simulink library "Custom_Valve_Choices_Lib"  (R2013a)
settings: Solver=ode45  SolverMode=SingleTasking  StartTime=0.0  StopTime=10.0  RelTol=1e-3
libraries: fl_lib x57, sh_lib x10, nesl_utility x8, Custom_Valve_Orifices_Lib x3, Custom_Valve_Choices_Lib x1
(part 1 of 2)
Description:
  | Copyright 2013 The MathWorks, Inc.
settings Model: Creator=smiller  LastModifiedBy=smiller

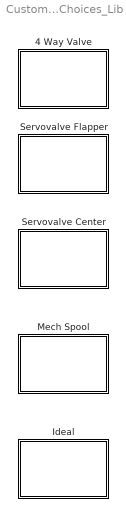
== system Custom_Valve_Choices_Lib ==
  4 Way Valve : Subsystem  BlockChoice=Ideal
      settings: TemplateBlock=self  MemberBlocks=Ideal,Mech Spool,Servovalve Center,Servovalve Flapper
      mask Display: disp(' ');
  Ideal : Subsystem  mask(Four-Way Valve){orifice_width=24.5, max_spool_travel=0.005, x0_orifice_PA=0, x0_orifice_PB=0, x0_orifice_AT=0, x0_orifice_BT=0}
      mask prompts: orifice_width "Orifice Width (mm):"; max_spool_travel "Max Orifice Length (m):"; x0_orifice_PA "Initial Opening PA (mm):"; x0_orifice_PB "Initial Opening PB (mm):"; x0_orifice_AT "Initial Opening AT (mm):"; x0_orifice_BT "Initial Opening BT (mm):"
      mask help: Four-way hydraulic directional valve.
      mask Display:
      | plot([0;337.311462499201;337.311462499201;0;0], [566.910021007061;566.910021007061;0;0;566.910021007061])
      | %hold on
      | plot([84.6585631370544;241.503668949008], [353;353])
      | plot([84.6585631370544;241.503668949008], [214;214])
      | plot([84.6585631370544;241.503668949008;241.503668949008;84.6585631370544;84.6585631370544], [491;491;76;76;491])
      | plot([84.6585631370544;241.503668949008], [449;449])
      | plot([241.503668949008;210.071657784283], [310;310])
      | plot([210.071657784283;210.071657784283;210.071657784283], [326;295;310.414731502533])
      | plot([241.503668949008;210.071657784283], [257;257])
      | plot([210.071657784283;210.071657784283;210.071657784283], [272;241;236.464468762279])
      | plot([84.6585631370544;115.964594297111], [257;257])
      | plot([115.964594297111;115.964594297111;115.964594297111], [272;241;236.464468762279])
      | plot([84.6585631370544;115.964594297111], [310;310])
      | plot([115.964594297111;115.964594297111;115.964594297111], [326;295;310.414731502533])
      | plot([84.6585631370544;241.503668949008], [185;110])
      | plot([241.503668949008;84.6585631370544], [185;110])
      | plot([84.6585631370544;241.503668949008], [395;395])
      | patch([85.0365031510592;110.547454096377;121.885654516518;85.0365031510592], [110;140;120;110], [0;0;0])
      | plot([85.0365031510592;110.547454096377;121.885654516518;85.0365031510592], [110;140;120;110])
      | patch([240.936758928001;204.087607562542;215.425807982683;240.936758928001], [109;120;140;109], [0;0;0])
      | plot([240.936758928001;204.087607562542;215.425807982683;240.936758928001], [109;120;140;109])
      | patch([83.6507230997086;127.554754726589;127.554754726589;83.6507230997086], [451;461;440;451], [0;0;0])
      | plot([83.6507230997086;127.554754726589;127.554754726589;83.6507230997086], [451;461;440;451])
      | patch([245.283069089055;201.253057457507;201.253057457507;245.283069089055], [394;405;384;394], [0;0;0])
      | plot([245.283069089055;201.253057457507;201.253057457507;245.283069089055], [394;405;384;394])
      | 
      | %plot([241.5; 241.5;201; 201], [491; 566; 566; 491])
      | %patch([241; 205; 222; 241], [525;525;495;525], [0;0;0]')
      | %plot([241.5; 241.5;201; 201], [76; 0; 0; 76])
      | %patch([241; 205; 222; 241], [40;40;70;40], [0;0;0])
      | %plot([241.5; 201], [11; 26])
      | %plot([241.5; 201], [561; 541])
      | 
      | %plot([127; 85;127; 85], [491; 511; 531; 551])
      | %plot([127; 85;127; 85], [76; 56; 36; 16])
      | %hold off
      | 
      | 
      | color('red');
      | port_label('LConn', 1,'A')
      | port_label('LConn', 2,'B')
      | port_label('RConn', 1,'S')
      | port_label('RConn', 2,'P')
      | port_label('RConn', 3,'T')
  Mech Spool : Subsystem  mask(Four-Way Valve with Spool){orifice_width=24.5, max_spool_travel=0.005, x0_orifice_PA=0, x0_orifice_PB=0, x0_orifice_AT=0, x0_orifice_BT=0, spool_mass=0.124, ctr_spr_stiffness=36000*100, spool_damping=324*10, spool_rad_clear=0.05}
      mask prompts: orifice_width "Orifice Width (mm):"; max_spool_travel "Max Orifice Length (m):"; x0_orifice_PA "Initial Opening PA (mm):"; x0_orifice_PB "Initial Opening PB (mm):"; x0_orifice_AT "Initial Opening AT (mm):"; x0_orifice_BT "Initial Opening BT (mm):"; spool_mass "Spool Mass (kg):"; ctr_spr_stiffness "Centering Spring Stiffness (N/m):"; spool_damping "Spool Damping (N/(m/s)):"; spool_rad_clear "Spool Radial Clearance (mm):"
      mask help: Four-way valve including mechanical model of spool. The spool is centered by a spring.
      mask Display:
      | plot([0;337.311462499201;337.311462499201;0;0], [566.910021007061;566.910021007061;0;0;566.910021007061])
      | %hold on
      | plot([84.6585631370544;241.503668949008], [353;353])
      | plot([84.6585631370544;241.503668949008], [214;214])
      | plot([84.6585631370544;241.503668949008;241.503668949008;84.6585631370544;84.6585631370544], [491;491;76;76;491])
      | plot([84.6585631370544;241.503668949008], [449;449])
      | plot([241.503668949008;210.071657784283], [310;310])
      | plot([210.071657784283;210.071657784283;210.071657784283], [326;295;310.414731502533])
      | plot([241.503668949008;210.071657784283], [257;257])
      | plot([210.071657784283;210.071657784283;210.071657784283], [272;241;236.464468762279])
      | plot([84.6585631370544;115.964594297111], [257;257])
      | plot([115.964594297111;115.964594297111;115.964594297111], [272;241;236.464468762279])
      | plot([84.6585631370544;115.964594297111], [310;310])
      | plot([115.964594297111;115.964594297111;115.964594297111], [326;295;310.414731502533])
      | plot([84.6585631370544;241.503668949008], [185;110])
      | plot([241.503668949008;84.6585631370544], [185;110])
      | plot([84.6585631370544;241.503668949008], [395;395])
      | patch([85.0365031510592;110.547454096377;121.885654516518;85.0365031510592], [110;140;120;110], [0;0;0])
      | plot([85.0365031510592;110.547454096377;121.885654516518;85.0365031510592], [110;140;120;110])
      | patch([240.936758928001;204.087607562542;215.425807982683;240.936758928001], [109;120;140;109], [0;0;0])
      | plot([240.936758928001;204.087607562542;215.425807982683;240.936758928001], [109;120;140;109])
      | patch([83.6507230997086;127.554754726589;127.554754726589;83.6507230997086], [451;461;440;451], [0;0;0])
      | plot([83.6507230997086;127.554754726589;127.554754726589;83.6507230997086], [451;461;440;451])
      | patch([245.283069089055;201.253057457507;201.253057457507;245.283069089055], [394;405;384;394], [0;0;0])
      | plot([245.283069089055;201.253057457507;201.253057457507;245.283069089055], [394;405;384;394])
      | 
      | plot([241.5; 241.5;201; 201], [491; 566; 566; 491])
      | %patch([241; 205; 222; 241], [525;525;495;525], [0;0;0]')
      | plot([241.5; 241.5;201; 201], [76; 0; 0; 76])
      | %patch([241; 205; 222; 241], [40;40;70;40], [0;0;0])
      | %plot([241.5; 201], [11; 26])
      | %plot([241.5; 201], [561; 541])
      | 
      | plot([127; 85;127; 85], [491; 511; 531; 551])
      | plot([127; 85;127; 85], [76; 56; 36; 16])
      | %hold off
      | 
      | 
      | color('cyan');
      | port_label('LConn', 1,'A')
      | port_label('LConn', 2,'B')
      | port_label('RConn', 1,'S')
      | port_label('RConn', 2,'P')
      | port_label('RConn', 3,'T')
  Servovalve Center : Subsystem  mask(Four-Way Servovalve, Centering Spring){orifice_width=24.5, max_spool_travel=0.005, x0_orifice_PA=0, x0_orifice_PB=0, x0_orifice_AT=0, x0_orifice_BT=0, spool_mass=0.124, ctr_spr_stiffness=3600000, spool_damping=162, spool_rad_clear=0.05, x0_nozzle=0.5, max_nozzle_area=3.14, pump_spool_orifice_area=1}
      mask prompts: orifice_width "Orifice Width (mm):"; max_spool_travel "Max Orifice Length (m):"; x0_orifice_PA "Initial Opening PA (mm):"; x0_orifice_PB "Initial Opening PB (mm):"; x0_orifice_AT "Initial Opening AT (mm):"; x0_orifice_BT "Initial Opening BT (mm):"; spool_mass "Spool Mass (kg):"; ctr_spr_stiffness "Centering Spring Stiffness (N/m):"; spool_damping "Spool Damping (N/(m/s)):"; spool_rad_clear "Spool Radial Clearance (mm):"; x0_nozzle "Nozzle Initial Opening (mm):"; max_nozzle_area "Nozzle Max Area (mm^2):"; pump_spool_orifice_area "Pump Spool Orifice Area (mm^2):"
      mask help: Four-way servovalve with electrical actuation of a flapper nozzle to control spool movement. The spool is centered by a spring.
      mask Display:
      | plot([0;337.311462499201;337.311462499201;0;0], [566.910021007061;566.910021007061;0;0;566.910021007061])
      | %hold on
      | plot([84.6585631370544;241.503668949008], [353;353])
      | plot([84.6585631370544;241.503668949008], [214;214])
      | plot([84.6585631370544;241.503668949008;241.503668949008;84.6585631370544;84.6585631370544], [491;491;76;76;491])
      | plot([84.6585631370544;241.503668949008], [449;449])
      | plot([241.503668949008;210.071657784283], [310;310])
      | plot([210.071657784283;210.071657784283;210.071657784283], [326;295;310.414731502533])
      | plot([241.503668949008;210.071657784283], [257;257])
      | plot([210.071657784283;210.071657784283;210.071657784283], [272;241;236.464468762279])
      | plot([84.6585631370544;115.964594297111], [257;257])
      | plot([115.964594297111;115.964594297111;115.964594297111], [272;241;236.464468762279])
      | plot([84.6585631370544;115.964594297111], [310;310])
      | plot([115.964594297111;115.964594297111;115.964594297111], [326;295;310.414731502533])
      | plot([84.6585631370544;241.503668949008], [185;110])
      | plot([241.503668949008;84.6585631370544], [185;110])
      | plot([84.6585631370544;241.503668949008], [395;395])
      | patch([85.0365031510592;110.547454096377;121.885654516518;85.0365031510592], [110;140;120;110], [0;0;0])
      | plot([85.0365031510592;110.547454096377;121.885654516518;85.0365031510592], [110;140;120;110])
      | patch([240.936758928001;204.087607562542;215.425807982683;240.936758928001], [109;120;140;109], [0;0;0])
      | plot([240.936758928001;204.087607562542;215.425807982683;240.936758928001], [109;120;140;109])
      | patch([83.6507230997086;127.554754726589;127.554754726589;83.6507230997086], [451;461;440;451], [0;0;0])
      | plot([83.6507230997086;127.554754726589;127.554754726589;83.6507230997086], [451;461;440;451])
      | patch([245.283069089055;201.253057457507;201.253057457507;245.283069089055], [394;405;384;394], [0;0;0])
      | plot([245.283069089055;201.253057457507;201.253057457507;245.283069089055], [394;405;384;394])
      | 
      | plot([241.5; 241.5;201; 201], [491; 566; 566; 491])
      | patch([241; 205; 222; 241], [525;525;495;525], [0;0;0]')
      | plot([241.5; 241.5;201; 201], [76; 0; 0; 76])
      | patch([241; 205; 222; 241], [40;40;70;40], [0;0;0])
      | %plot([241.5; 201], [11; 26])
      | %plot([241.5; 201], [561; 541])
      | 
      | plot([127; 85;127; 85], [491; 511; 531; 551])
      | plot([127; 85;127; 85], [76; 56; 36; 16])
      | %hold off
      | 
      | ;color('orange');
      | port_label('LConn', 1,'A')
      | port_label('LConn', 2,'B')
      | port_label('RConn', 1,'S')
      | port_label('RConn', 2,'P')
      | port_label('RConn', 3,'T')
  Servovalve Flapper : Subsystem  mask(Four-Way Servovalve, Flapper-Spool){orifice_width=24.5, max_spool_travel=0.005, x0_orifice_PA=0, x0_orifice_PB=0, x0_orifice_AT=0, x0_orifice_BT=0, spool_mass=0.124, spool_damping=162, spool_rad_clear=0.05, x0_nozzle=0.5, max_nozzle_area=3.14, pump_spool_orifice_area=1}
      mask prompts: orifice_width "Orifice Width (mm):"; max_spool_travel "Max Orifice Length (m):"; x0_orifice_PA "Initial Opening PA (mm):"; x0_orifice_PB "Initial Opening PB (mm):"; x0_orifice_AT "Initial Opening AT (mm):"; x0_orifice_BT "Initial Opening BT (mm):"; spool_mass "Spool Mass (kg):"; spool_damping "Centering Spring Damping (N/(m/s)):"; spool_rad_clear "Spool Radial Clearance (mm):"; x0_nozzle "Nozzle Initial Opening (mm):"; max_nozzle_area "Nozzle Max Area (mm^2):"; pump_spool_orifice_area "Pump Spool Orifice Area (mm):"
      mask help: Four-way servovalve with electrical actuation of a flapper-nozzle to control spool movement. The flapper is connected mechanically to spool.
      mask Display:
      | plot([0;337.311462499201;337.311462499201;0;0], [566.910021007061;566.910021007061;0;0;566.910021007061])
      | %hold on
      | plot([84.6585631370544;241.503668949008], [353;353])
      | plot([84.6585631370544;241.503668949008], [214;214])
      | plot([84.6585631370544;241.503668949008;241.503668949008;84.6585631370544;84.6585631370544], [491;491;76;76;491])
      | plot([84.6585631370544;241.503668949008], [449;449])
      | plot([241.503668949008;210.071657784283], [310;310])
      | plot([210.071657784283;210.071657784283;210.071657784283], [326;295;310.414731502533])
      | plot([241.503668949008;210.071657784283], [257;257])
      | plot([210.071657784283;210.071657784283;210.071657784283], [272;241;236.464468762279])
      | plot([84.6585631370544;115.964594297111], [257;257])
      | plot([115.964594297111;115.964594297111;115.964594297111], [272;241;236.464468762279])
      | plot([84.6585631370544;115.964594297111], [310;310])
      | plot([115.964594297111;115.964594297111;115.964594297111], [326;295;310.414731502533])
      | plot([84.6585631370544;241.503668949008], [185;110])
      | plot([241.503668949008;84.6585631370544], [185;110])
      | plot([84.6585631370544;241.503668949008], [395;395])
      | patch([85.0365031510592;110.547454096377;121.885654516518;85.0365031510592], [110;140;120;110], [0;0;0])
      | plot([85.0365031510592;110.547454096377;121.885654516518;85.0365031510592], [110;140;120;110])
      | patch([240.936758928001;204.087607562542;215.425807982683;240.936758928001], [109;120;140;109], [0;0;0])
      | plot([240.936758928001;204.087607562542;215.425807982683;240.936758928001], [109;120;140;109])
      | patch([83.6507230997086;127.554754726589;127.554754726589;83.6507230997086], [451;461;440;451], [0;0;0])
      | plot([83.6507230997086;127.554754726589;127.554754726589;83.6507230997086], [451;461;440;451])
      | patch([245.283069089055;201.253057457507;201.253057457507;245.283069089055], [394;405;384;394], [0;0;0])
      | plot([245.283069089055;201.253057457507;201.253057457507;245.283069089055], [394;405;384;394])
      | 
      | plot([241.5; 241.5;201; 201], [491; 566; 566; 491])
      | patch([241; 205; 222; 241], [525;525;495;525], [0;0;0]')
      | plot([241.5; 241.5;201; 201], [76; 0; 0; 76])
      | patch([241; 205; 222; 241], [40;40;70;40], [0;0;0])
      | %plot([241.5; 201], [11; 26])
      | %plot([241.5; 201], [561; 541])
      | 
      | %plot([127; 85;127; 85], [491; 511; 531; 551])
      | %plot([127; 85;127; 85], [76; 56; 36; 16])
      | %hold off
      | 
      | 
      | color('green');
      | port_label('LConn', 1,'A')
      | port_label('LConn', 2,'B')
      | port_label('RConn', 1,'S')
      | port_label('RConn', 2,'P')
      | port_label('RConn', 3,'T')

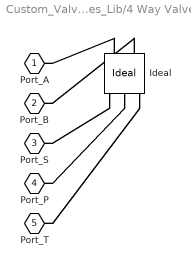
== system Custom_Valve_Choices_Lib/4 Way Valve ==
  Ideal : Custom_Valve_Choices_Lib/Ideal  orifice_width=24.5  max_spool_travel=0.005  x0_orifice_PA=0  x0_orifice_PB=0  x0_orifice_AT=0  x0_orifice_BT=0
  Port_A : PMIOPort  Port=1  Side=Left
  Port_B : PMIOPort  Port=2  Side=Left
  Port_S : PMIOPort  Port=3  Side=Right
  Port_P : PMIOPort  Port=4  Side=Right
  Port_T : PMIOPort  Port=5  Side=Right
  connections:
  Ideal/LConn1 -- Port_A/RConn1
  Ideal/LConn2 -- Port_B/RConn1
  Ideal/RConn1 -- Port_S/RConn1
  Ideal/RConn2 -- Port_P/RConn1
  Ideal/RConn3 -- Port_T/RConn1

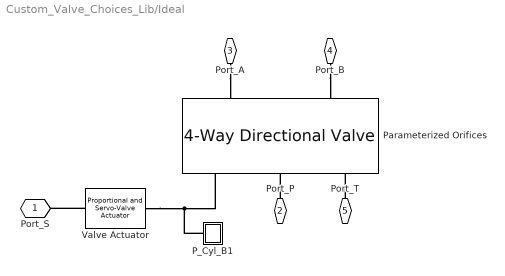
== system Custom_Valve_Choices_Lib/Ideal ==
  P_Cyl_B1 : Subsystem
  Parameterized Orifices : sh_lib/Valves/Directional Valves/4-Way Directional Valve  mdl_type=1  area_max=orifice_width*max_spool_travel*1e3 mm^2  opening_max=max_spool_travel m  opening_tab="[  -0.002 0 0.002 0.005 0.015 ] m"  area_tab="[  1e-09 2.0352e-07 4.0736e-05 0.00011438 0.00034356 ] m^2"  pressure_tab="[  -1e+07 -5e+06 -2e+06 2e+06 5e+06 1e+07 ] Pa"  flow_rate_tab="[  -1e-07 -7.0711e-08 -4.4721e-08 4.4721e-08 7.0711e-08 1e-07 ; -2.0352e-05 -1.4391e-05 -9.1017e-06 9.1017e-06 1.4391e-05 2.0352e-05 ; -0.0040736 -0.0028805 -0.0018218 0.0018218 0.0028805 0.0040736 ; -0.011438 -0.0080879 -0.0051152 0.0051152 0.0080879 0.011438 ; -0.034356 -0.024293 -0.015364 0.015364 0.024293 0.034356 ; ] m^3/s"  interp_method=1  extrap_method=1  C_d=0.7  x_0_P_A=x0_orifice_PA mm  x_0_P_B=x0_orifice_PB mm  x_0_A_T=x0_orifice_AT mm  x_0_B_T=x0_orifice_BT mm  Re_cr=12  A_leak=1e-12 m^2  LocalVarLogging=[]
  Valve Actuator : sh_lib/Valves/Valve Actuators/Proportional and Servo-Valve Actuator  gain=250  time_constant=1e-2 s  saturation=0.3  LocalVarLogging=[]
  Port_S : PMIOPort  Port=1  Side=Right
  Port_P : PMIOPort  Port=2  Side=Right
  Port_A : PMIOPort  Port=3  Side=Left
  Port_B : PMIOPort  Port=4  Side=Left
  Port_T : PMIOPort  Port=5  Side=Right
  connections:
  Valve Actuator/LConn1 -- Port_S/RConn1
  Port_T/RConn1 -- Parameterized Orifices/RConn3
  Port_P/RConn1 -- Parameterized Orifices/RConn2
  Parameterized Orifices/RConn1 -- P_Cyl_B1/LConn1 -- Valve Actuator/RConn1
  Port_B/RConn1 -- Parameterized Orifices/LConn2
  Port_A/RConn1 -- Parameterized Orifices/LConn1

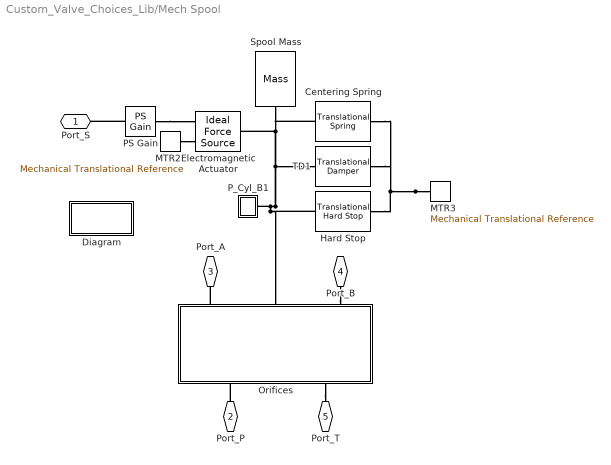
== system Custom_Valve_Choices_Lib/Mech Spool ==
  Centering Spring : fl_lib/Mechanical/Translational Elements/Translational Spring  Tag=Factory Generic  spr_rate=ctr_spr_stiffness N/m  init_def=0 m  f_Log=off  v_Log=off  x_Log=off  LocalVarNames=|force|deformation  LocalVarDescs=|Spring force (N)|Spring deformation (m)  LocalVarLogging=[0 0]
  Diagram : Subsystem
      mask Display: image(imread('Custom_Valve_Proportional_Spool.jpg'));
  Electromagnetic Actuator : fl_lib/Mechanical/Mechanical Sources/Ideal Force Source  Tag=Factory Generic  v_Log=off  f_Log=off  LocalVarNames=|force|rel_velocity|power  LocalVarDescs=|Force (N)|Relative velocity (m/s)|Power generated by the source (W)  LocalVarLogging=[0 0 0]
  Hard Stop : fl_lib/Mechanical/Translational Elements/Translational Hard Stop  Tag=Factory Generic  upper_bnd=max_spool_travel m  lower_bnd=-max_spool_travel m  stiff_up=1e+06 N/m  stiff_low=1e+06 N/m  D_up=150 N/(m/s)  D_low=150 N/(m/s)  initial_position=0 m  f_Log=off  v_Log=off  x_Log=off  LocalVarNames=|contact_force|rel_displacement  LocalVarDescs=|Contact force (N)|Slider-case relative displacement (m)  LocalVarLogging=[0 0]
  MTR2 : fl_lib/Mechanical/Translational Elements/Mechanical Translational Reference  Tag=Factory Generic  f_Log=off  LocalVarNames=|f  LocalVarDescs=|f  LocalVarLogging=[]
  MTR3 : fl_lib/Mechanical/Translational Elements/Mechanical Translational Reference  Tag=Factory Generic  f_Log=off  LocalVarNames=|f  LocalVarDescs=|f  LocalVarLogging=[]
  Orifices : Subsystem  BlockChoice=No Force
      link override No Force: or_width=orifice_width  x0_PA=x0_orifice_PA  x0_PB=x0_orifice_PB  x0_AT=x0_orifice_AT  x0_BT=x0_orifice_BT
      link override Parameterized: or_width=orifice_width  x0_PA=x0_orifice_PA  x0_PB=x0_orifice_PA  x0_AT=x0_orifice_PA  x0_BT=x0_orifice_PA  max_sp_trv=max_spool_travel
      link override With Force: or_width=orifice_width  x0_PA=x0_orifice_PA  x0_PB=x0_orifice_PB  x0_AT=x0_orifice_AT  x0_BT=x0_orifice_BT  rad_clearance=spool_rad_clear
      settings: AttributesFormatString=%<BlockChoice>  TemplateBlock=Custom_Valve_Orifices_Lib/Orifices  MemberBlocks=No Force,Parameterized,With Force
  PS Gain : fl_lib/Physical Signals/Functions/PS Gain  gain=5e4*100  LocalVarLogging=[]
  P_Cyl_B1 : Subsystem
  Spool Mass : fl_lib/Mechanical/Translational Elements/Mass  Tag=Factory Generic  mass=spool_mass kg  initial_velocity=0 m/s  f_Log=off  LocalVarNames=|force|velocity  LocalVarDescs=|Inertia force (N)|Mass absolute velocity (m/s)  LocalVarLogging=[0 0]
  TD1 : fl_lib/Mechanical/Translational Elements/Translational Damper  Tag=Factory Generic  D=spool_damping N/(m/s)  f_Log=off  v_Log=off  LocalVarNames=|force|rel_velocity|power  LocalVarDescs=|Damping force (N)|Damper relative velocity (m/s)|Power dissipated in the damper (W)  LocalVarLogging=[0 0 0]
  Port_S : PMIOPort  Port=1  Side=Right
  Port_P : PMIOPort  Port=2  Side=Right
  Port_A : PMIOPort  Port=3  Side=Left
  Port_B : PMIOPort  Port=4  Side=Left
  Port_T : PMIOPort  Port=5  Side=Right
  connections:
  Port_P/RConn1 -- Orifices/LConn1
  Orifices/RConn1 -- Port_A/RConn1
  Port_B/RConn1 -- Orifices/RConn3
  P_Cyl_B1/LConn1 -- Electromagnetic Actuator/LConn1 -- Spool Mass/LConn1 -- Centering Spring/LConn1 -- TD1/LConn1 -- Hard Stop/LConn1 -- Orifices/RConn2
  Orifices/LConn2 -- Port_T/RConn1
  MTR3/LConn1 -- Hard Stop/RConn1 -- Centering Spring/RConn1 -- TD1/RConn1
  PS Gain/RConn1 -- Electromagnetic Actuator/RConn1
  PS Gain/LConn1 -- Port_S/RConn1
  MTR2/LConn1 -- Electromagnetic Actuator/RConn2

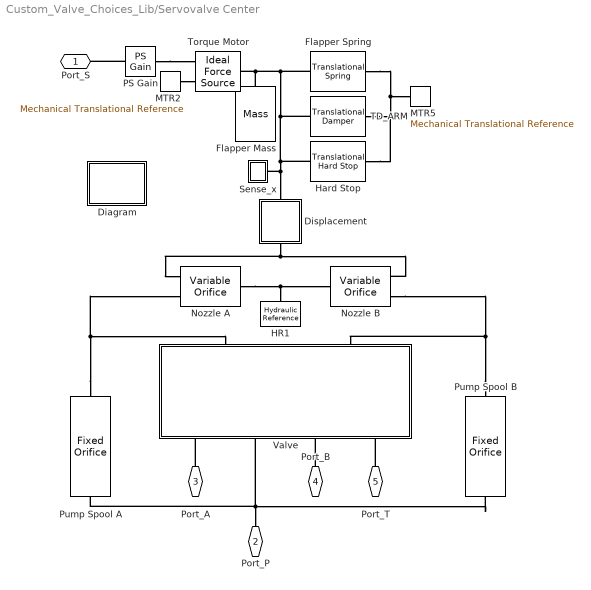
== system Custom_Valve_Choices_Lib/Servovalve Center ==
  Diagram : Subsystem
      mask Display: image(imread('Custom_Valve_Servovalve_Spring_Centered.jpg'));
  Displacement : Subsystem
      mask Display:
      | plot([311.800511553884;0;0;311.800511553884;311.800511553884], [311.800511553884;311.800511553884;0;0;311.800511553884])
      | plot([25.5109509453177;56.6910021007061;70.8637526258826;96.3747035712004;127.554754726589;155.900255776942;184.245756827295;212.591257877648;235.26765871793;252.274959348142;283.455010503531], [155.900255776942;155.900255776942;110.547454096377;198.418507352471;113.382004201412;198.418507352471;116.216554306448;198.418507352471;113.382004201412;155.900255776942;155.900255776942])
      | plot([155.900255776942;155.900255776942], [266.447709873319;198.418507352471])
      | patch([155.900255776942;170.073006302118;141.727505251765;155.900255776942], [198.418507352471;226.764008402824;226.764008402824;198.418507352471], [0;0;0])
      | plot([155.900255776942;170.073006302118;141.727505251765;155.900255776942], [198.418507352471;226.764008402824;226.764008402824;198.418507352471])
  Flapper Mass : fl_lib/Mechanical/Translational Elements/Mass  Tag=Factory Generic  mass=0.012 kg  initial_velocity=0 m/s  f_Log=off  LocalVarNames=|force|velocity  LocalVarDescs=|Inertia force (N)|Mass absolute velocity (m/s)  LocalVarLogging=[0 0]
  Flapper Spring : fl_lib/Mechanical/Translational Elements/Translational Spring  Tag=Factory Generic  spr_rate=150000 N/m  init_def=0 m  f_Log=off  v_Log=off  x_Log=off  LocalVarNames=|force|deformation  LocalVarDescs=|Spring force (N)|Spring deformation (m)  LocalVarLogging=[0 0]
  HR1 : fl_lib/Hydraulic/Hydraulic Elements/Hydraulic Reference  Tag=Factory Generic  q_Log=off  LocalVarNames=|q  LocalVarDescs=|q  LocalVarLogging=[]
  Hard Stop : fl_lib/Mechanical/Translational Elements/Translational Hard Stop  Tag=Factory Generic  upper_bnd=x0_nozzle mm  lower_bnd=-x0_nozzle mm  stiff_up=1e+06 N/m  stiff_low=1e+06 N/m  D_up=150 N/(m/s)  D_low=150 N/(m/s)  initial_position=0 m  f_Log=off  v_Log=off  x_Log=off  LocalVarNames=|contact_force|rel_displacement  LocalVarDescs=|Contact force (N)|Slider-case relative displacement (m)  LocalVarLogging=[0 0]
  MTR2 : fl_lib/Mechanical/Translational Elements/Mechanical Translational Reference  Tag=Factory Generic  f_Log=off  LocalVarNames=|f  LocalVarDescs=|f  LocalVarLogging=[]
  MTR5 : fl_lib/Mechanical/Translational Elements/Mechanical Translational Reference  Tag=Factory Generic  f_Log=off  LocalVarNames=|f  LocalVarDescs=|f  LocalVarLogging=[]
  Nozzle A : sh_lib/Orifices/Variable Orifice  Tag=Factory Generic  mdl_type=1  area_max=max_nozzle_area mm^2  opening_max=2*x0_nozzle mm  opening_tab="[  -0.002 0 0.005 0.015 ] m"  area_tab="[  1e-12 4e-12 1e-05 1.02e-05 ] m^2"  pressure_tab="[  -5e+06 -2e+06 2e+06 5e+06 ] Pa"  flow_rate_tab="[  -1e-12 -6e-14 6e+12 1e+11 ; -8e-08 -4e-08 4e+06 8e+06 ; -0.0025 -0.00103 0.001 0.0024 ; -0.00258 -0.001032 0.00106 0.00247 ; ] m^3/s"  interp_method=1  extrap_method=1  or=1  C_d=0.7  x_0=x0_nozzle mm  Re_cr=12  A_leak=1e-9 m^2  flow_rate_Log=off  pr_drop_Log=off  Re_Log=off  orif_opening_Log=off  power_Log=off  LocalVarNames=|flow_rate|pr_drop|Re|orif_opening|power  LocalVarDescs=|Flow rate through the orifice (m^3)|Pressure drop across the orifice (Pa)|Reynolds number|Orifice opening (m)|Power dissipated in the orifice (W)  LocalVarLogging=[0 0 0 0 0]
  Nozzle B : sh_lib/Orifices/Variable Orifice  Tag=Factory Generic  mdl_type=1  area_max=max_nozzle_area mm^2  opening_max=2*x0_nozzle mm  opening_tab="[  -0.002 0 0.005 0.015 ] m"  area_tab="[  1e-12 4e-12 1e-05 1.02e-05 ] m^2"  pressure_tab="[  -5e+06 -2e+06 2e+06 5e+06 ] Pa"  flow_rate_tab="[  -1e-12 -6e-14 6e+12 1e+11 ; -8e-08 -4e-08 4e+06 8e+06 ; -0.0025 -0.00103 0.001 0.0024 ; -0.00258 -0.001032 0.00106 0.00247 ; ] m^3/s"  interp_method=1  extrap_method=1  or=2  C_d=0.7  x_0=x0_nozzle mm  Re_cr=12  A_leak=1e-9 m^2  flow_rate_Log=off  pr_drop_Log=off  Re_Log=off  orif_opening_Log=off  power_Log=off  LocalVarNames=|flow_rate|pr_drop|Re|orif_opening|power  LocalVarDescs=|Flow rate through the orifice (m^3)|Pressure drop across the orifice (Pa)|Reynolds number|Orifice opening (m)|Power dissipated in the orifice (W)  LocalVarLogging=[0 0 0 0 0]
  PS Gain : fl_lib/Physical Signals/Functions/PS Gain  gain=-5e4  LocalVarLogging=[]
  "Pump Spool A " : sh_lib/Orifices/Fixed Orifice  Tag=Factory Generic  area=pump_spool_orifice_area mm^2  C_d=0.7  Re_cr=12  flow_rate_Log=off  pr_drop_Log=off  Re_Log=off  power_Log=off  LocalVarNames=|flow_rate|pr_drop|Re|power  LocalVarDescs=|Flow rate through the orifice (m^3/s)|Pressure drop across the orifice (Pa)|Reynolds number|Power (W)  LocalVarLogging=[0 0 0 0]
  Pump Spool B : sh_lib/Orifices/Fixed Orifice  Tag=Factory Generic  area=pump_spool_orifice_area mm^2  C_d=0.7  Re_cr=12  flow_rate_Log=off  pr_drop_Log=off  Re_Log=off  power_Log=off  LocalVarNames=|flow_rate|pr_drop|Re|power  LocalVarDescs=|Flow rate through the orifice (m^3/s)|Pressure drop across the orifice (Pa)|Reynolds number|Power (W)  LocalVarLogging=[0 0 0 0]
  Sense_x : Subsystem
  TD_ARM : fl_lib/Mechanical/Translational Elements/Translational Damper  Tag=Factory Generic  D=25 N/(m/s)  f_Log=off  v_Log=off  LocalVarNames=|force|rel_velocity|power  LocalVarDescs=|Damping force (N)|Damper relative velocity (m/s)|Power dissipated in the damper (W)  LocalVarLogging=[0 0 0]
  Torque Motor : fl_lib/Mechanical/Mechanical Sources/Ideal Force Source  Tag=Factory Generic  v_Log=off  f_Log=off  LocalVarNames=|force|rel_velocity|power  LocalVarDescs=|Force (N)|Relative velocity (m/s)|Power generated by the source (W)  LocalVarLogging=[0 0 0]
  Valve : Subsystem
  Port_S : PMIOPort  Port=1  Side=Right
  Port_P : PMIOPort  Port=2  Side=Right
  Port_A : PMIOPort  Port=3  Side=Left
  Port_B : PMIOPort  Port=4  Side=Left
  Port_T : PMIOPort  Port=5  Side=Right
  connections:
  Port_T/RConn1 -- Valve/RConn4
  Port_B/RConn1 -- Valve/RConn3
  Port_A/RConn1 -- Valve/RConn1
  PS Gain/RConn1 -- Torque Motor/RConn1
  PS Gain/LConn1 -- Port_S/RConn1
  Hard Stop/LConn1 -- Displacement/LConn1 -- Sense_x/LConn1 -- TD_ARM/LConn1 -- Flapper Spring/LConn1 -- Flapper Mass/LConn1 -- Torque Motor/LConn1
  Displacement/RConn1 -- Nozzle B/LConn1 -- Nozzle A/LConn1
  Pump Spool B/LConn1 -- "Pump Spool A "/LConn1 -- Port_P/RConn1 -- Valve/RConn2
  Flapper Spring/RConn1 -- MTR5/LConn1 -- Hard Stop/RConn1 -- TD_ARM/RConn1
  Nozzle A/RConn1 -- HR1/LConn1 -- Nozzle B/RConn1
  "Pump Spool A "/RConn1 -- Nozzle A/LConn2 -- Valve/LConn1
  Pump Spool B/RConn1 -- Nozzle B/LConn2 -- Valve/LConn2
  MTR2/LConn1 -- Torque Motor/RConn2

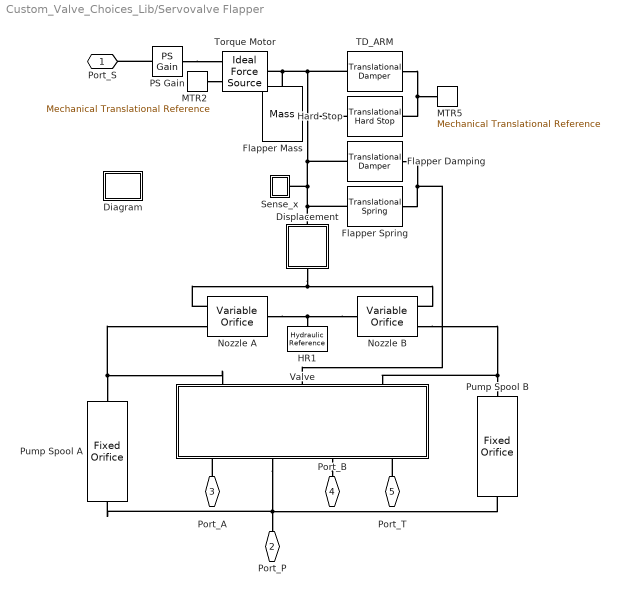
== system Custom_Valve_Choices_Lib/Servovalve Flapper ==
  Diagram : Subsystem
      mask Display: image(imread('Custom_Valve_Servovalve_Feedback.jpg'));
  Displacement : Subsystem
      mask Display:
      | plot([311.800511553884;0;0;311.800511553884;311.800511553884], [311.800511553884;311.800511553884;0;0;311.800511553884])
      | plot([25.5109509453177;56.6910021007061;70.8637526258826;96.3747035712004;127.554754726589;155.900255776942;184.245756827295;212.591257877648;235.26765871793;252.274959348142;283.455010503531], [155.900255776942;155.900255776942;110.547454096377;198.418507352471;113.382004201412;198.418507352471;116.216554306448;198.418507352471;113.382004201412;155.900255776942;155.900255776942])
      | plot([155.900255776942;155.900255776942], [266.447709873319;198.418507352471])
      | patch([155.900255776942;170.073006302118;141.727505251765;155.900255776942], [198.418507352471;226.764008402824;226.764008402824;198.418507352471], [0;0;0])
      | plot([155.900255776942;170.073006302118;141.727505251765;155.900255776942], [198.418507352471;226.764008402824;226.764008402824;198.418507352471])
  Flapper Damping : fl_lib/Mechanical/Translational Elements/Translational Damper  Tag=Factory Generic  D=250 N/(m/s)  f_Log=off  v_Log=off  LocalVarNames=|force|rel_velocity|power  LocalVarDescs=|Damping force (N)|Damper relative velocity (m/s)|Power dissipated in the damper (W)  LocalVarLogging=[0 0 0]
  Flapper Mass : fl_lib/Mechanical/Translational Elements/Mass  Tag=Factory Generic  mass=0.012 kg  initial_velocity=0 m/s  f_Log=off  LocalVarNames=|force|velocity  LocalVarDescs=|Inertia force (N)|Mass absolute velocity (m/s)  LocalVarLogging=[0 0]
  Flapper Spring : fl_lib/Mechanical/Translational Elements/Translational Spring  Tag=Factory Generic  spr_rate=6000 N/m  init_def=0 m  f_Log=off  v_Log=off  x_Log=off  LocalVarNames=|force|deformation  LocalVarDescs=|Spring force (N)|Spring deformation (m)  LocalVarLogging=[0 0]
  HR1 : fl_lib/Hydraulic/Hydraulic Elements/Hydraulic Reference  Tag=Factory Generic  q_Log=off  LocalVarNames=|q  LocalVarDescs=|q  LocalVarLogging=[]
  Hard Stop : fl_lib/Mechanical/Translational Elements/Translational Hard Stop  Tag=Factory Generic  upper_bnd=x0_nozzle mm  lower_bnd=-x0_nozzle mm  stiff_up=1e+06 N/m  stiff_low=1e+06 N/m  D_up=150 N/(m/s)  D_low=150 N/(m/s)  initial_position=0 m  f_Log=off  v_Log=off  x_Log=off  LocalVarNames=|contact_force|rel_displacement  LocalVarDescs=|Contact force (N)|Slider-case relative displacement (m)  LocalVarLogging=[0 0]
  MTR2 : fl_lib/Mechanical/Translational Elements/Mechanical Translational Reference  Tag=Factory Generic  f_Log=off  LocalVarNames=|f  LocalVarDescs=|f  LocalVarLogging=[]
  MTR5 : fl_lib/Mechanical/Translational Elements/Mechanical Translational Reference  Tag=Factory Generic  f_Log=off  LocalVarNames=|f  LocalVarDescs=|f  LocalVarLogging=[]
  Nozzle A : sh_lib/Orifices/Variable Orifice  Tag=Factory Generic  mdl_type=1  area_max=max_nozzle_area mm^2  opening_max=2*x0_nozzle mm  opening_tab="[  -0.002 0 0.005 0.015 ] m"  area_tab="[  1e-12 4e-12 1e-05 1.02e-05 ] m^2"  pressure_tab="[  -5e+06 -2e+06 2e+06 5e+06 ] Pa"  flow_rate_tab="[  -1e-12 -6e-14 6e+12 1e+11 ; -8e-08 -4e-08 4e+06 8e+06 ; -0.0025 -0.00103 0.001 0.0024 ; -0.00258 -0.001032 0.00106 0.00247 ; ] m^3/s"  interp_method=1  extrap_method=1  or=1  C_d=0.7  x_0=x0_nozzle mm  Re_cr=12  A_leak=1e-9 m^2  flow_rate_Log=off  pr_drop_Log=off  Re_Log=off  orif_opening_Log=off  power_Log=off  LocalVarNames=|flow_rate|pr_drop|Re|orif_opening|power  LocalVarDescs=|Flow rate through the orifice (m^3)|Pressure drop across the orifice (Pa)|Reynolds number|Orifice opening (m)|Power dissipated in the orifice (W)  LocalVarLogging=[0 0 0 0 0]
  Nozzle B : sh_lib/Orifices/Variable Orifice  Tag=Factory Generic  mdl_type=1  area_max=max_nozzle_area mm^2  opening_max=2*x0_nozzle mm  opening_tab="[  -0.002 0 0.005 0.015 ] m"  area_tab="[  1e-12 4e-12 1e-05 1.02e-05 ] m^2"  pressure_tab="[  -5e+06 -2e+06 2e+06 5e+06 ] Pa"  flow_rate_tab="[  -1e-12 -6e-14 6e+12 1e+11 ; -8e-08 -4e-08 4e+06 8e+06 ; -0.0025 -0.00103 0.001 0.0024 ; -0.00258 -0.001032 0.00106 0.00247 ; ] m^3/s"  interp_method=1  extrap_method=1  or=2  C_d=0.7  x_0=x0_nozzle mm  Re_cr=12  A_leak=1e-9 m^2  flow_rate_Log=off  pr_drop_Log=off  Re_Log=off  orif_opening_Log=off  power_Log=off  LocalVarNames=|flow_rate|pr_drop|Re|orif_opening|power  LocalVarDescs=|Flow rate through the orifice (m^3)|Pressure drop across the orifice (Pa)|Reynolds number|Orifice opening (m)|Power dissipated in the orifice (W)  LocalVarLogging=[0 0 0 0 0]
  PS Gain : fl_lib/Physical Signals/Functions/PS Gain  gain=-3e4  LocalVarLogging=[]
  "Pump Spool A " : sh_lib/Orifices/Fixed Orifice  Tag=Factory Generic  area=pump_spool_orifice_area mm^2  C_d=0.7  Re_cr=12  flow_rate_Log=off  pr_drop_Log=off  Re_Log=off  power_Log=off  LocalVarNames=|flow_rate|pr_drop|Re|power  LocalVarDescs=|Flow rate through the orifice (m^3/s)|Pressure drop across the orifice (Pa)|Reynolds number|Power (W)  LocalVarLogging=[0 0 0 0]
  Pump Spool B : sh_lib/Orifices/Fixed Orifice  Tag=Factory Generic  area=pump_spool_orifice_area mm^2  C_d=0.7  Re_cr=12  flow_rate_Log=off  pr_drop_Log=off  Re_Log=off  power_Log=off  LocalVarNames=|flow_rate|pr_drop|Re|power  LocalVarDescs=|Flow rate through the orifice (m^3/s)|Pressure drop across the orifice (Pa)|Reynolds number|Power (W)  LocalVarLogging=[0 0 0 0]
  Sense_x : Subsystem
  TD_ARM : fl_lib/Mechanical/Translational Elements/Translational Damper  Tag=Factory Generic  D=25 N/(m/s)  f_Log=off  v_Log=off  LocalVarNames=|force|rel_velocity|power  LocalVarDescs=|Damping force (N)|Damper relative velocity (m/s)|Power dissipated in the damper (W)  LocalVarLogging=[0 0 0]
  Torque Motor : fl_lib/Mechanical/Mechanical Sources/Ideal Force Source  Tag=Factory Generic  v_Log=off  f_Log=off  LocalVarNames=|force|rel_velocity|power  LocalVarDescs=|Force (N)|Relative velocity (m/s)|Power generated by the source (W)  LocalVarLogging=[0 0 0]
  Valve : Subsystem
  Port_S : PMIOPort  Port=1  Side=Right
  Port_P : PMIOPort  Port=2  Side=Right
  Port_A : PMIOPort  Port=3  Side=Left
  Port_B : PMIOPort  Port=4  Side=Left
  Port_T : PMIOPort  Port=5  Side=Right
  connections:
  Port_A/RConn1 -- Valve/RConn1
  Valve/RConn3 -- Port_B/RConn1
  Port_T/RConn1 -- Valve/RConn4
  MTR2/LConn1 -- Torque Motor/RConn2
  Nozzle B/LConn2 -- Pump Spool B/RConn1 -- Valve/LConn3
  Valve/LConn1 -- Nozzle A/LConn2 -- "Pump Spool A "/RConn1
  Nozzle B/RConn1 -- HR1/LConn1 -- Nozzle A/RConn1
  Hard Stop/RConn1 -- MTR5/LConn1 -- TD_ARM/RConn1
  "Pump Spool A "/LConn1 -- Valve/RConn2 -- Pump Spool B/LConn1 -- Port_P/RConn1
  Flapper Spring/RConn1 -- Flapper Damping/RConn1 -- Valve/LConn2
  Displacement/RConn1 -- Nozzle B/LConn1 -- Nozzle A/LConn1
  Sense_x/LConn1 -- TD_ARM/LConn1 -- Torque Motor/LConn1 -- Flapper Mass/LConn1 -- Hard Stop/LConn1 -- Flapper Damping/LConn1 -- Flapper Spring/LConn1 -- Displacement/LConn1
  PS Gain/LConn1 -- Port_S/RConn1
  PS Gain/RConn1 -- Torque Motor/RConn1

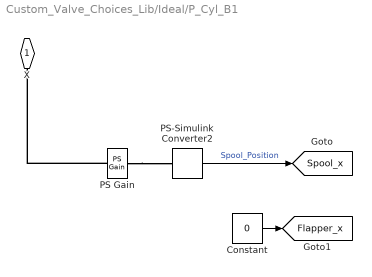
== system Custom_Valve_Choices_Lib/Ideal/P_Cyl_B1 ==
  Constant : Constant  Value=0
  PS Gain : fl_lib/Physical Signals/Functions/PS Gain  gain=1e3  LocalVarLogging=[]
  PS-Simulink Converter2 : nesl_utility/PS-Simulink Converter  PhysicalDomain=network_engine_domain  LeftPortType=input  RightPortType=output  SubClassName=ps_output  PseudoPeriodic=off  Frequencies=[]  Unit=mm  AffineConversion=off
  X : PMIOPort  Port=1  Side=Left
  tag scope: Flapper_x=global, Spool_x=global
  wires:
  PS-Simulink Converter2/1 -> [Spool_x]  "Spool_Position"
  Constant/1 -> [Flapper_x]
  connections:
  PS Gain/LConn1 -- X/RConn1
  PS Gain/RConn1 -- PS-Simulink Converter2/LConn1

== system Custom_Valve_Choices_Lib/Mech Spool/Diagram ==
  Diagram : Subsystem
      mask Display: image(imread('Custom_Valve_Proportional_Spool.jpg'));

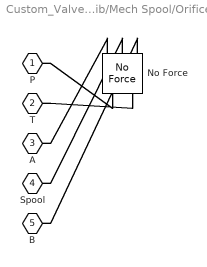
== system Custom_Valve_Choices_Lib/Mech Spool/Orifices ==
  No Force : Custom_Valve_Orifices_Lib/No Force  or_width=orifice_width  x0_PA=x0_orifice_PA  x0_PB=x0_orifice_PB  x0_AT=x0_orifice_AT  x0_BT=x0_orifice_BT
  P : PMIOPort  Port=1  Side=Left
  T : PMIOPort  Port=2  Side=Left
  A : PMIOPort  Port=3  Side=Right
  Spool : PMIOPort  Port=4  Side=Right
  B : PMIOPort  Port=5  Side=Right
  connections:
  No Force/LConn1 -- P/RConn1
  No Force/LConn2 -- T/RConn1
  No Force/RConn1 -- A/RConn1
  No Force/RConn2 -- Spool/RConn1
  No Force/RConn3 -- B/RConn1

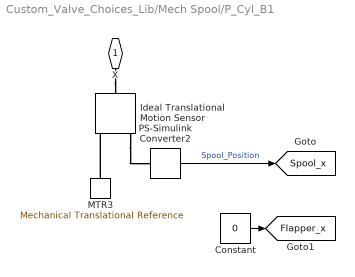
== system Custom_Valve_Choices_Lib/Mech Spool/P_Cyl_B1 ==
  Constant : Constant  Value=0
  Ideal Translational Motion Sensor : fl_lib/Mechanical/Mechanical Sensors/Ideal Translational Motion Sensor  Tag=Factory Generic  offset=0 m  v_Log=off  f_Log=off  x_Log=off  LocalVarNames=|v|f|x  LocalVarDescs=|v|f|x  LocalVarLogging=[]
  MTR3 : fl_lib/Mechanical/Translational Elements/Mechanical Translational Reference  Tag=Factory Generic  f_Log=off  LocalVarNames=|f  LocalVarDescs=|f  LocalVarLogging=[]
  PS-Simulink Converter2 : nesl_utility/PS-Simulink Converter  PhysicalDomain=network_engine_domain  LeftPortType=input  RightPortType=output  SubClassName=ps_output  PseudoPeriodic=off  Frequencies=[]  Unit=mm  AffineConversion=off
  X : PMIOPort  Port=1  Side=Left
  tag scope: Flapper_x=global, Spool_x=global
  wires:
  PS-Simulink Converter2/1 -> [Spool_x]  "Spool_Position"
  Constant/1 -> [Flapper_x]
  connections:
  MTR3/LConn1 -- Ideal Translational Motion Sensor/RConn1
  X/RConn1 -- Ideal Translational Motion Sensor/LConn1
  Ideal Translational Motion Sensor/RConn3 -- PS-Simulink Converter2/LConn1

== system Custom_Valve_Choices_Lib/Servovalve Center/Diagram ==
  Diagram : Subsystem
      mask Display: image(imread('Custom_Valve_Servovalve_Spring_Centered.jpg'));

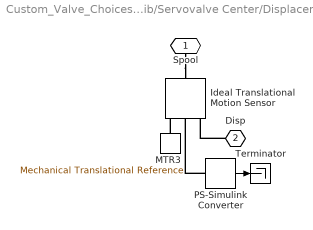
== system Custom_Valve_Choices_Lib/Servovalve Center/Displacement ==
  Ideal Translational Motion Sensor : fl_lib/Mechanical/Mechanical Sensors/Ideal Translational Motion Sensor  Tag=Factory Generic  offset=0 m  v_Log=off  f_Log=off  x_Log=off  LocalVarNames=|v|f|x  LocalVarDescs=|v|f|x  LocalVarLogging=[]
  MTR3 : fl_lib/Mechanical/Translational Elements/Mechanical Translational Reference  Tag=Factory Generic  f_Log=off  LocalVarNames=|f  LocalVarDescs=|f  LocalVarLogging=[]
  PS-Simulink Converter : nesl_utility/PS-Simulink Converter  PhysicalDomain=network_engine_domain  LeftPortType=input  RightPortType=output  SubClassName=ps_output  PseudoPeriodic=off  Frequencies=[]  Unit=1  AffineConversion=off
  Terminator : Terminator
  Spool : PMIOPort  Port=1  Side=Left
  Disp : PMIOPort  Port=2  Side=Right
  wires:
  PS-Simulink Converter/1 -> Terminator/1
  connections:
  MTR3/LConn1 -- Ideal Translational Motion Sensor/RConn1
  PS-Simulink Converter/LConn1 -- Ideal Translational Motion Sensor/RConn2
  Spool/RConn1 -- Ideal Translational Motion Sensor/LConn1
  Disp/RConn1 -- Ideal Translational Motion Sensor/RConn3

== system Custom_Valve_Choices_Lib/Servovalve Center/Sense_x ==
  Ideal Translational Motion Sensor : fl_lib/Mechanical/Mechanical Sensors/Ideal Translational Motion Sensor  Tag=Factory Generic  offset=0 m  v_Log=off  f_Log=off  x_Log=off  LocalVarNames=|v|f|x  LocalVarDescs=|v|f|x  LocalVarLogging=[]
  MTR3 : fl_lib/Mechanical/Translational Elements/Mechanical Translational Reference  Tag=Factory Generic  f_Log=off  LocalVarNames=|f  LocalVarDescs=|f  LocalVarLogging=[]
  PS-Simulink Converter2 : nesl_utility/PS-Simulink Converter  PhysicalDomain=network_engine_domain  LeftPortType=input  RightPortType=output  SubClassName=ps_output  PseudoPeriodic=off  Frequencies=[]  Unit=1  AffineConversion=off
  X : PMIOPort  Port=1  Side=Left
  tag scope: Flapper_x=global
  wires:
  PS-Simulink Converter2/1 -> [Flapper_x]  "Flapper_Position"
  connections:
  Ideal Translational Motion Sensor/RConn3 -- PS-Simulink Converter2/LConn1
  X/RConn1 -- Ideal Translational Motion Sensor/LConn1
  MTR3/LConn1 -- Ideal Translational Motion Sensor/RConn1

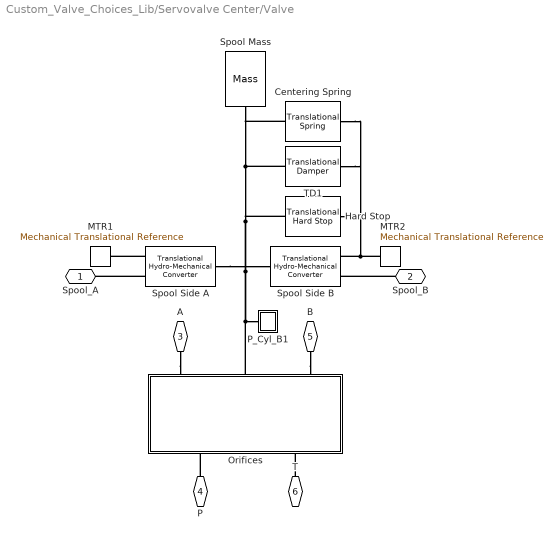
== system Custom_Valve_Choices_Lib/Servovalve Center/Valve ==
  Centering Spring : fl_lib/Mechanical/Translational Elements/Translational Spring  Tag=Factory Generic  spr_rate=ctr_spr_stiffness N/m  init_def=0 m  f_Log=off  v_Log=off  x_Log=off  LocalVarNames=|force|deformation  LocalVarDescs=|Spring force (N)|Spring deformation (m)  LocalVarLogging=[0 0]
  Hard Stop : fl_lib/Mechanical/Translational Elements/Translational Hard Stop  Tag=Factory Generic  upper_bnd=max_spool_travel m  lower_bnd=-max_spool_travel m  stiff_up=1e+06 N/m  stiff_low=1e+06 N/m  D_up=150 N/(m/s)  D_low=150 N/(m/s)  initial_position=0 m  f_Log=off  v_Log=off  x_Log=off  LocalVarNames=|contact_force|rel_displacement  LocalVarDescs=|Contact force (N)|Slider-case relative displacement (m)  LocalVarLogging=[0 0]
  MTR1 : fl_lib/Mechanical/Translational Elements/Mechanical Translational Reference  Tag=Factory Generic  f_Log=off  LocalVarNames=|f  LocalVarDescs=|f  LocalVarLogging=[]
  MTR2 : fl_lib/Mechanical/Translational Elements/Mechanical Translational Reference  Tag=Factory Generic  f_Log=off  LocalVarNames=|f  LocalVarDescs=|f  LocalVarLogging=[]
  Orifices : Subsystem  BlockChoice=No Force
      link override No Force: or_width=orifice_width  x0_PA=x0_orifice_PA  x0_PB=x0_orifice_PB  x0_AT=x0_orifice_AT  x0_BT=x0_orifice_BT
      link override Parameterized: or_width=orifice_width  x0_PA=x0_orifice_PA  x0_PB=x0_orifice_PB  x0_AT=x0_orifice_AT  x0_BT=x0_orifice_BT  max_sp_trv=max_spool_travel
      link override With Force: or_width=orifice_width  x0_PA=x0_orifice_PA  x0_PB=x0_orifice_PB  x0_AT=x0_orifice_AT  x0_BT=x0_orifice_BT  rad_clearance=spool_rad_clear
      settings: AttributesFormatString=%<BlockChoice>  TemplateBlock=Custom_Valve_Orifices_Lib/Orifices  MemberBlocks=No Force,Parameterized,With Force
  P_Cyl_B1 : Subsystem
  Spool Mass : fl_lib/Mechanical/Translational Elements/Mass  Tag=Factory Generic  mass=spool_mass kg  initial_velocity=0 m/s  f_Log=off  LocalVarNames=|force|velocity  LocalVarDescs=|Inertia force (N)|Mass absolute velocity (m/s)  LocalVarLogging=[0 0]
  Spool Side A : fl_lib/Hydraulic/Hydraulic Elements/Translational Hydro-Mechanical Converter  Tag=Factory Generic  area=78 mm^2  or=1  dir=1  f_Log=off  q_Log=off  LocalVarNames=|flow_rate|pressure|force|power  LocalVarDescs=|Flow rate into the chamber (m^3/s)|Pressure at the inlet (Pa)|Output force (N)|Power (W)  LocalVarLogging=[0 0 0 0]
  Spool Side B : fl_lib/Hydraulic/Hydraulic Elements/Translational Hydro-Mechanical Converter  Tag=Factory Generic  area=78 mm^2  or=2  dir=1  f_Log=off  q_Log=off  LocalVarNames=|flow_rate|pressure|force|power  LocalVarDescs=|Flow rate into the chamber (m^3/s)|Pressure at the inlet (Pa)|Output force (N)|Power (W)  LocalVarLogging=[0 0 0 0]
  TD1 : fl_lib/Mechanical/Translational Elements/Translational Damper  Tag=Factory Generic  D=spool_damping N/(m/s)  f_Log=off  v_Log=off  LocalVarNames=|force|rel_velocity|power  LocalVarDescs=|Damping force (N)|Damper relative velocity (m/s)|Power dissipated in the damper (W)  LocalVarLogging=[0 0 0]
  Spool_A : PMIOPort  Port=1  Side=Left
  Spool_B : PMIOPort  Port=2  Side=Left
  A : PMIOPort  Port=3  Side=Right
  P : PMIOPort  Port=4  Side=Right
  B : PMIOPort  Port=5  Side=Right
  T : PMIOPort  Port=6  Side=Right
  connections:
  T/RConn1 -- Orifices/LConn2
  P/RConn1 -- Orifices/LConn1
  B/RConn1 -- Orifices/RConn3
  A/RConn1 -- Orifices/RConn1
  Orifices/RConn2 -- P_Cyl_B1/LConn1 -- Spool Side A/RConn1 -- Spool Side B/RConn1 -- Hard Stop/LConn1 -- TD1/LConn1 -- Centering Spring/LConn1 -- Spool Mass/LConn1
  Spool Side A/LConn1 -- MTR1/LConn1
  Spool Side A/LConn2 -- Spool_A/RConn1
  Spool_B/RConn1 -- Spool Side B/LConn2
  Hard Stop/RConn1 -- Centering Spring/RConn1 -- TD1/RConn1 -- Spool Side B/LConn1 -- MTR2/LConn1

== system Custom_Valve_Choices_Lib/Servovalve Flapper/Diagram ==
  Diagram : Subsystem
      mask Display: image(imread('Custom_Valve_Servovalve_Feedback.jpg'));

== system Custom_Valve_Choices_Lib/Servovalve Flapper/Displacement ==
  Ideal Translational Motion Sensor : fl_lib/Mechanical/Mechanical Sensors/Ideal Translational Motion Sensor  Tag=Factory Generic  offset=0 m  v_Log=off  f_Log=off  x_Log=off  LocalVarNames=|v|f|x  LocalVarDescs=|v|f|x  LocalVarLogging=[]
  MTR3 : fl_lib/Mechanical/Translational Elements/Mechanical Translational Reference  Tag=Factory Generic  f_Log=off  LocalVarNames=|f  LocalVarDescs=|f  LocalVarLogging=[]
  PS-Simulink Converter : nesl_utility/PS-Simulink Converter  PhysicalDomain=network_engine_domain  LeftPortType=input  RightPortType=output  SubClassName=ps_output  PseudoPeriodic=off  Frequencies=[]  Unit=1  AffineConversion=off
  Terminator : Terminator
  Spool : PMIOPort  Port=1  Side=Left
  Disp : PMIOPort  Port=2  Side=Right
  wires:
  PS-Simulink Converter/1 -> Terminator/1
  connections:
  MTR3/LConn1 -- Ideal Translational Motion Sensor/RConn1
  PS-Simulink Converter/LConn1 -- Ideal Translational Motion Sensor/RConn2
  Spool/RConn1 -- Ideal Translational Motion Sensor/LConn1
  Disp/RConn1 -- Ideal Translational Motion Sensor/RConn3

== system Custom_Valve_Choices_Lib/Servovalve Flapper/Sense_x ==
  Ideal Translational Motion Sensor : fl_lib/Mechanical/Mechanical Sensors/Ideal Translational Motion Sensor  Tag=Factory Generic  offset=0 m  v_Log=off  f_Log=off  x_Log=off  LocalVarNames=|v|f|x  LocalVarDescs=|v|f|x  LocalVarLogging=[]
  MTR3 : fl_lib/Mechanical/Translational Elements/Mechanical Translational Reference  Tag=Factory Generic  f_Log=off  LocalVarNames=|f  LocalVarDescs=|f  LocalVarLogging=[]
  PS-Simulink Converter2 : nesl_utility/PS-Simulink Converter  PhysicalDomain=network_engine_domain  LeftPortType=input  RightPortType=output  SubClassName=ps_output  PseudoPeriodic=off  Frequencies=[]  Unit=1  AffineConversion=off
  X : PMIOPort  Port=1  Side=Left
  tag scope: Flapper_x=global
  wires:
  PS-Simulink Converter2/1 -> [Flapper_x]  "Flapper_Position"
  connections:
  Ideal Translational Motion Sensor/RConn3 -- PS-Simulink Converter2/LConn1
  X/RConn1 -- Ideal Translational Motion Sensor/LConn1
  MTR3/LConn1 -- Ideal Translational Motion Sensor/RConn1

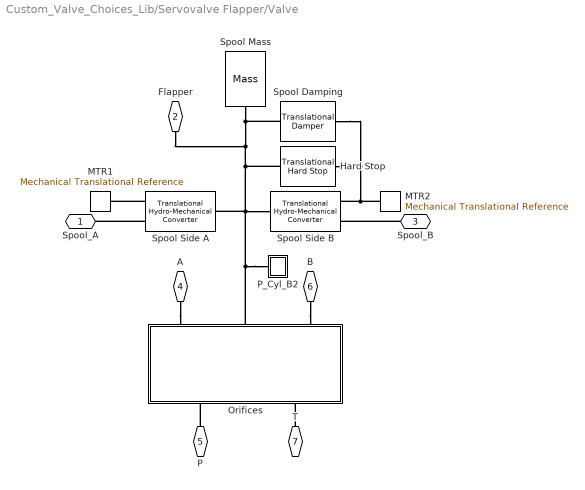
== system Custom_Valve_Choices_Lib/Servovalve Flapper/Valve ==
  Hard Stop : fl_lib/Mechanical/Translational Elements/Translational Hard Stop  Tag=Factory Generic  upper_bnd=max_spool_travel m  lower_bnd=-max_spool_travel m  stiff_up=1e+06 N/m  stiff_low=1e+06 N/m  D_up=150 N/(m/s)  D_low=150 N/(m/s)  initial_position=0 m  f_Log=off  v_Log=off  x_Log=off  LocalVarNames=|contact_force|rel_displacement  LocalVarDescs=|Contact force (N)|Slider-case relative displacement (m)  LocalVarLogging=[0 0]
  MTR1 : fl_lib/Mechanical/Translational Elements/Mechanical Translational Reference  Tag=Factory Generic  f_Log=off  LocalVarNames=|f  LocalVarDescs=|f  LocalVarLogging=[]
  MTR2 : fl_lib/Mechanical/Translational Elements/Mechanical Translational Reference  Tag=Factory Generic  f_Log=off  LocalVarNames=|f  LocalVarDescs=|f  LocalVarLogging=[]
  Orifices : Subsystem  BlockChoice=With Force
      link override No Force: or_width=orifice_width  x0_PA=x0_orifice_PA  x0_PB=x0_orifice_PB  x0_AT=x0_orifice_AT  x0_BT=x0_orifice_BT
      link override Parameterized: or_width=orifice_width  x0_PA=x0_orifice_PA  x0_PB=x0_orifice_PB  x0_AT=x0_orifice_AT  x0_BT=x0_orifice_BT  max_sp_trv=max_spool_travel
      link override With Force: or_width=orifice_width  x0_PA=x0_orifice_PA  x0_PB=x0_orifice_PB  x0_AT=x0_orifice_AT  x0_BT=x0_orifice_BT  rad_clearance=spool_rad_clear
      settings: AttributesFormatString=%<BlockChoice>  TemplateBlock=Custom_Valve_Orifices_Lib/Orifices  MemberBlocks=No Force,Parameterized,With Force
  P_Cyl_B2 : Subsystem
  Spool Damping : fl_lib/Mechanical/Translational Elements/Translational Damper  Tag=Factory Generic  D=spool_damping N/(m/s)  f_Log=off  v_Log=off  LocalVarNames=|force|rel_velocity|power  LocalVarDescs=|Damping force (N)|Damper relative velocity (m/s)|Power dissipated in the damper (W)  LocalVarLogging=[0 0 0]
  Spool Mass : fl_lib/Mechanical/Translational Elements/Mass  Tag=Factory Generic  mass=spool_mass kg  initial_velocity=0 m/s  f_Log=off  LocalVarNames=|force|velocity  LocalVarDescs=|Inertia force (N)|Mass absolute velocity (m/s)  LocalVarLogging=[0 0]
  Spool Side A : fl_lib/Hydraulic/Hydraulic Elements/Translational Hydro-Mechanical Converter  Tag=Factory Generic  area=78 mm^2  or=1  dir=1  f_Log=off  q_Log=off  LocalVarNames=|flow_rate|pressure|force|power  LocalVarDescs=|Flow rate into the chamber (m^3/s)|Pressure at the inlet (Pa)|Output force (N)|Power (W)  LocalVarLogging=[0 0 0 0]
  Spool Side B : fl_lib/Hydraulic/Hydraulic Elements/Translational Hydro-Mechanical Converter  Tag=Factory Generic  area=78 mm^2  or=2  dir=1  f_Log=off  q_Log=off  LocalVarNames=|flow_rate|pressure|force|power  LocalVarDescs=|Flow rate into the chamber (m^3/s)|Pressure at the inlet (Pa)|Output force (N)|Power (W)  LocalVarLogging=[0 0 0 0]
  Spool_A : PMIOPort  Port=1  Side=Left
  Flapper : PMIOPort  Port=2  Side=Left
  Spool_B : PMIOPort  Port=3  Side=Left
  A : PMIOPort  Port=4  Side=Right
  P : PMIOPort  Port=5  Side=Right
  B : PMIOPort  Port=6  Side=Right
  T : PMIOPort  Port=7  Side=Right
  connections:
  T/RConn1 -- Orifices/LConn2
  A/RConn1 -- Orifices/RConn1
  P/RConn1 -- Orifices/LConn1
  B/RConn1 -- Orifices/RConn3
  MTR2/LConn1 -- Hard Stop/RConn1 -- Spool Damping/RConn1 -- Spool Side B/LConn1
  Spool_B/RConn1 -- Spool Side B/LConn2
  Spool Side A/LConn2 -- Spool_A/RConn1
  Spool Side A/LConn1 -- MTR1/LConn1
  P_Cyl_B2/LConn1 -- Spool Side A/RConn1 -- Spool Side B/RConn1 -- Flapper/RConn1 -- Spool Mass/LConn1 -- Spool Damping/LConn1 -- Hard Stop/LConn1 -- Orifices/RConn2

== system Custom_Valve_Choices_Lib/Mech Spool/Diagram/Diagram ==

== system Custom_Valve_Choices_Lib/Servovalve Center/Diagram/Diagram ==
